simulink model "KSimulator_robotExM1_NPC"  (Simulink 8.9)
settings: Solver=FixedStepDiscrete  StartTime=0.0  StopTime=5  FixedStep=0.01  RelTol=1e-3  EnableMultiTasking=on
undefined symbols (not defined in the file or in its folder): SimpleRobotPlot
settings Model: SuppressorTable=22 serialization::archive 11 0 6 0 0 0 11 0  Creator=E. Dean  LastModifiedBy=dean
settings OptimizationCC: ExpressionDepthLimit=2147483647
settings DebuggingCC: SolverPrmCheckMsg=warning

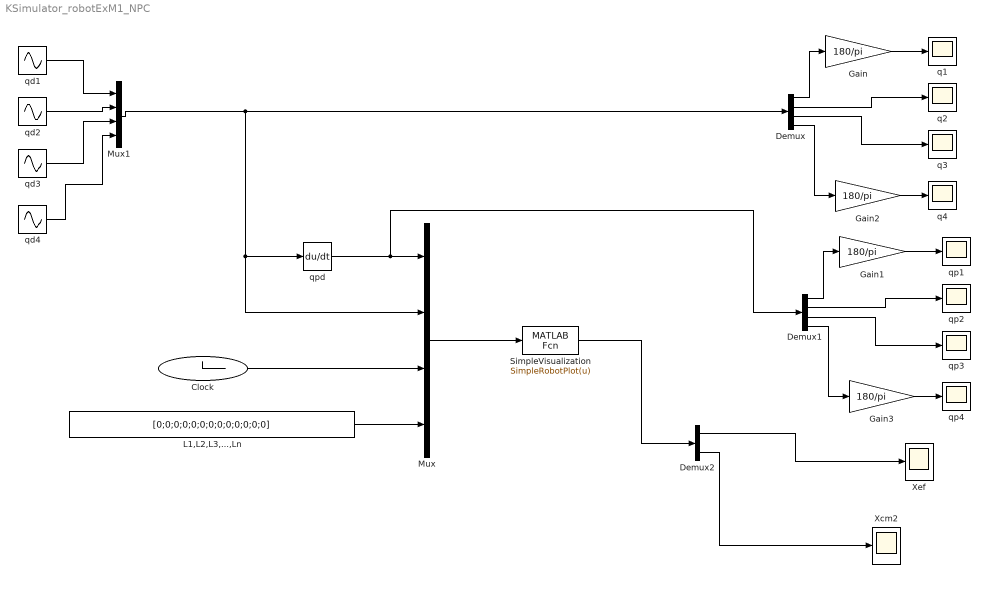
== system KSimulator_robotExM1_NPC ==
  Clock : Clock
  Demux : Demux
  Demux1 : Demux
  Demux2 : Demux  Outputs=2
  Gain{,1..3} (4 alike) : Gain  Gain=180/pi
  L1,L2,L3,...,Ln : Constant  Value=[0;0;0;0;0;0;0;0;0;0;0;0;0]
  Mux : Mux
  Mux1 : Mux
  SimpleVisualization : MATLABFcn  MATLABFcn=SimpleRobotPlot(u)  OutputDimensions=6
  Xcm2 : Scope
  Xef : Scope
  q{1..4} (4 alike) : Scope
  qd1 : Sin  Amplitude=0.5  SampleTime=0
  qd2 : Sin  Amplitude=0.3  Bias=0.3  SampleTime=0
  qd3 : Sin  Amplitude=pi  SampleTime=0
  qd4 : Sin  Amplitude=pi  SampleTime=0
  qp{1..4} (4 alike) : Scope
  qpd : Derivative
  wires:
  Demux/2 -> q2/1
  Mux/1 -> SimpleVisualization/1
  Demux/3 -> q3/1
  qd1/1 -> Mux1/1
  qd2/1 -> Mux1/2
  qd3/1 -> Mux1/3
  Mux1/1 -> qpd/1, Mux/2, Demux/1
  qpd/1 -> Demux1/1, Mux/1
  SimpleVisualization/1 -> Demux2/1
  Demux2/1 -> Xef/1
  Demux2/2 -> Xcm2/1
  qd4/1 -> Mux1/4
  Demux/1 -> Gain/1
  Gain/1 -> q1/1
  Gain2/1 -> q4/1
  Demux/4 -> Gain2/1
  Demux1/1 -> Gain1/1
  Gain3/1 -> qp4/1
  Gain1/1 -> qp1/1
  Demux1/2 -> qp2/1
  Demux1/4 -> Gain3/1
  Demux1/3 -> qp3/1
  Clock/1 -> Mux/3
  L1,L2,L3,...,Ln/1 -> Mux/4
